simulink model "RGB_GRAY"  (R2016a)
settings: Solver=VariableStepAuto  StartTime=0.0  StopTime=10.0  RelTol=1e-3
undefined symbols (not defined in the file or in its folder): Rec, SDTV
libraries: visionsources x2, visionconversions x1
settings Model: Creator=Auroshis  LastModifiedBy=Auroshis

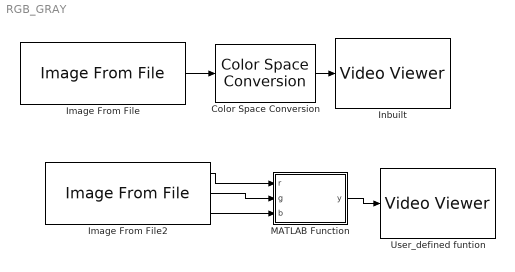
== system RGB_GRAY ==
  Color Space Conversion : visionconversions/Color Space  Conversion  conversion=Obsolete  conversionActive=R'G'B' to intensity  wp_str=D65  rec=Rec. 601 (SDTV)  sys=1125/60/2:1  imagePorts=One multidimensional signal
  Image From File : visionsources/Image From File  Tag=vipblks_nd  FileName=peppers.png  imagePorts=One multidimensional signal  Ts=0.1  ImageDataType=Inherit from input image  Signed=on  WordLength=16  sdImageDataType=uint(8)  FractionLengthMode=User-defined  FractionLength=15  OutPortLabels=R|G|B
  Image From File2 : visionsources/Image From File  Tag=vipblks_nd  FileName=peppers.png  imagePorts=Separate color signals  Ts=0.1  ImageDataType=Inherit from input image  Signed=on  WordLength=16  sdImageDataType=uint(8)  FractionLengthMode=User-defined  FractionLength=15  OutPortLabels=R|G|B
  Inbuilt : VideoViewer  Tag=addition  FigPos=[351.4 642.8 409.6 300]
  MATLAB Function : MATLAB Function  TreatAsAtomicUnit=on
  User_defined funtion : VideoViewer  Tag=addition  FigPos=[761 644.4 409.6 300]
  wires:
  Image From File/1 -> Color Space Conversion/1
  Color Space Conversion/1 -> Inbuilt/1
  Image From File2/1 -> MATLAB Function/1(r)
  MATLAB Function/1(y) -> User_defined funtion/1
  Image From File2/2 -> MATLAB Function/2(g)
  Image From File2/3 -> MATLAB Function/3(b)

== matlab function RGB_GRAY/MATLAB Function ==
  data: r input; y output; g input; b input
function y = fcn(r,g,b)
y = 0.2989*r + 0.5870*g + 0.1140*b;
